simulink model "q2_part_c_continous"  (R2020b)
settings: Solver=VariableStepAuto  StartTime=0.0  StopTime=10  RelTol=1e-3
model workspace (MATLAB code in the model file):
  | G11 = tf(tfs.NUM(1,1),tfs.DEN(1,1),Ts);
  | G12 = tf(tfs.NUM(2,1),tfs.DEN(2,1),Ts);
  | G13 = tf(tfs.NUM(3,1),tfs.DEN(3,1),Ts);
  | G21 = tf(tfs.NUM(1,2),tfs.DEN(1,2),Ts);
  | G22 = tf(tfs.NUM(2,2),tfs.DEN(2,2),Ts);
  | G23 = tf(tfs.NUM(3,2),tfs.DEN(3,2),Ts);
values from neighbouring files (symbols this model uses):
  tfs = tf(sys)    [q2_a_and_b.m]
  Ts = tout(2) - tout(1)    [q2_a_and_b.m]
libraries: cstblocks x6
settings Model: OrderedModelArguments=off  Creator=Jamesh  LastModifiedBy=HP

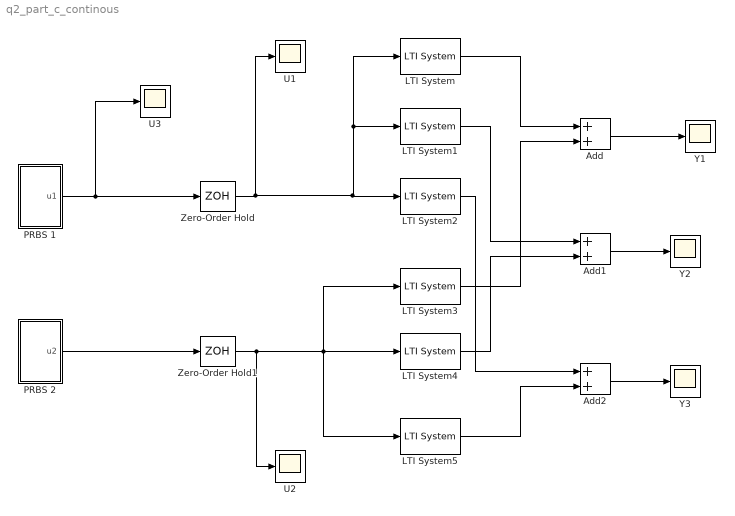
== system q2_part_c_continous ==
  Add : Sum
  Add1 : Sum
  Add2 : Sum
  LTI System : cstblocks/LTI System  sys=G11  IC=[]
  LTI System1 : cstblocks/LTI System  sys=G12  IC=[]
  LTI System2 : cstblocks/LTI System  sys=G13  IC=[]
  LTI System3 : cstblocks/LTI System  sys=G21  IC=[]
  LTI System4 : cstblocks/LTI System  sys=G22  IC=[]
  LTI System5 : cstblocks/LTI System  sys=G23  IC=[]
  PRBS 1 : Subsystem
  PRBS 2 : Subsystem
  U1 : Scope
  U2 : Scope
  U3 : Scope
  Y1 : Scope
  Y2 : Scope
  Y3 : Scope
  Zero-Order Hold : ZeroOrderHold  SampleTime=-1
  Zero-Order Hold1 : ZeroOrderHold  SampleTime=-1
  wires:
  LTI System/1 -> Add/1
  LTI System3/1 -> Add/2
  LTI System1/1 -> Add1/1
  LTI System4/1 -> Add1/2
  LTI System2/1 -> Add2/1
  LTI System5/1 -> Add2/2
  Add1/1 -> Y2/1
  Add/1 -> Y1/1
  Add2/1 -> Y3/1
  PRBS 1/1(u1) -> U3/1, Zero-Order Hold/1
  Zero-Order Hold/1 -> LTI System2/1, LTI System1/1, LTI System/1, U1/1
  Zero-Order Hold1/1 -> U2/1, LTI System3/1, LTI System5/1, LTI System4/1
  PRBS 2/1(u2) -> Zero-Order Hold1/1

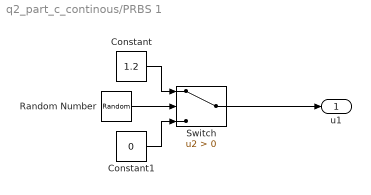
== system q2_part_c_continous/PRBS 1 ==
  Constant : Constant  Value=1.2
  Constant1 : Constant  Value=0
  Random Number : RandomNumber  Seed=1  SampleTime=0.25
  Switch : Switch  Criteria=u2 > Threshold
  u1 : Outport
  wires:
  Switch/1 -> u1/1
  Random Number/1 -> Switch/2
  Constant1/1 -> Switch/3
  Constant/1 -> Switch/1

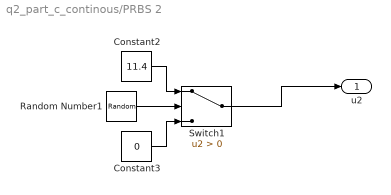
== system q2_part_c_continous/PRBS 2 ==
  Constant2 : Constant  Value=11.4
  Constant3 : Constant  Value=0
  Random Number1 : RandomNumber  Seed=2  SampleTime=0.25
  Switch1 : Switch  Criteria=u2 > Threshold
  u2 : Outport
  wires:
  Random Number1/1 -> Switch1/2
  Switch1/1 -> u2/1
  Constant3/1 -> Switch1/3
  Constant2/1 -> Switch1/1
